simulink model "feedback_yaw"  (R2018b)
settings: Solver=VariableStepAuto  StartTime=0.0  StopTime=10  RelTol=1e-3
undefined symbols (not defined in the file): Ayaw, Ayaw_prime, Byaw, Byaw_prime, Cyaw, Cyaw_prime, Dyaw, Dyaw_prime, Kyaw, Syaw, x0_chap, x0yaw
settings Model: Creator=Rafik  LastModifiedBy=Rafik

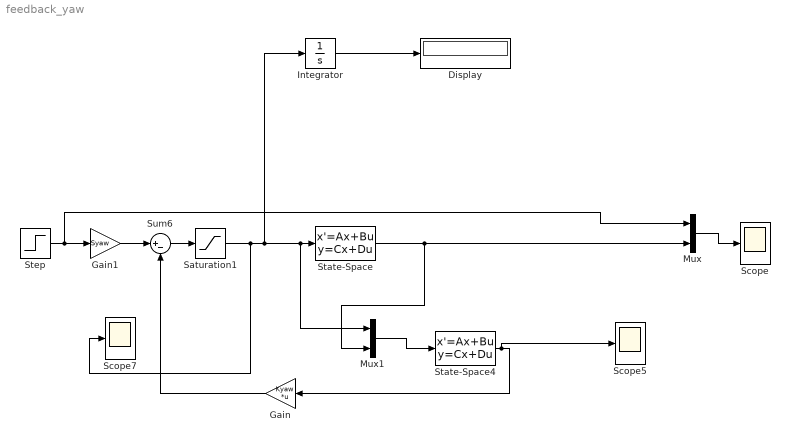
== system feedback_yaw ==
  Display : Display
  Gain : Gain  Gain=Kyaw  Multiplication=Matrix(K*u)
  Gain1 : Gain  Gain=Syaw
  Integrator : Integrator
  Mux : Mux  Inputs=2
  Mux1 : Mux  Inputs=2
  Saturation1 : Saturate  UpperLimit=110  LowerLimit=-110
  Scope : Scope
  Scope5 : Scope
  Scope7 : Scope
  State-Space : StateSpace  A=Ayaw  B=Byaw  C=Cyaw  D=Dyaw  InitialCondition=x0yaw
  State-Space4 : StateSpace  A=Ayaw_prime  B=Byaw_prime  C=Cyaw_prime  D=Dyaw_prime  InitialCondition=x0_chap
  Step : Step  Time=0  After=0.5  SampleTime=0
  Sum6 : Sum  Inputs=|+-
  wires:
  Sum6/1 -> Saturation1/1
  Mux1/1 -> State-Space4/1
  Step/1 -> Mux/1, Gain1/1
  Gain1/1 -> Sum6/1
  Gain/1 -> Sum6/2
  State-Space4/1 -> Scope5/1, Gain/1
  State-Space/1 -> Mux/2, Mux1/2
  Mux/1 -> Scope/1
  Saturation1/1 -> Integrator/1, Mux1/1, State-Space/1, Scope7/1
  Integrator/1 -> Display/1
